simulink model "BergmanModelExtended"  (R2020b)
settings: Solver=VariableStepAuto  StartTime=0.0  StopTime=1000  RelTol=1e-3
undefined symbols (not defined in the file): U1, u3
settings Model: Creator=marti  LastModifiedBy=13234
settings DataIOCC: ReturnWorkspaceOutputs=off
settings DebuggingCC: ArithmeticOperatorsInVariantConditions=warning
settings SFSimCC: CustomCodeUndefinedFunction=UseInterfaceOnly

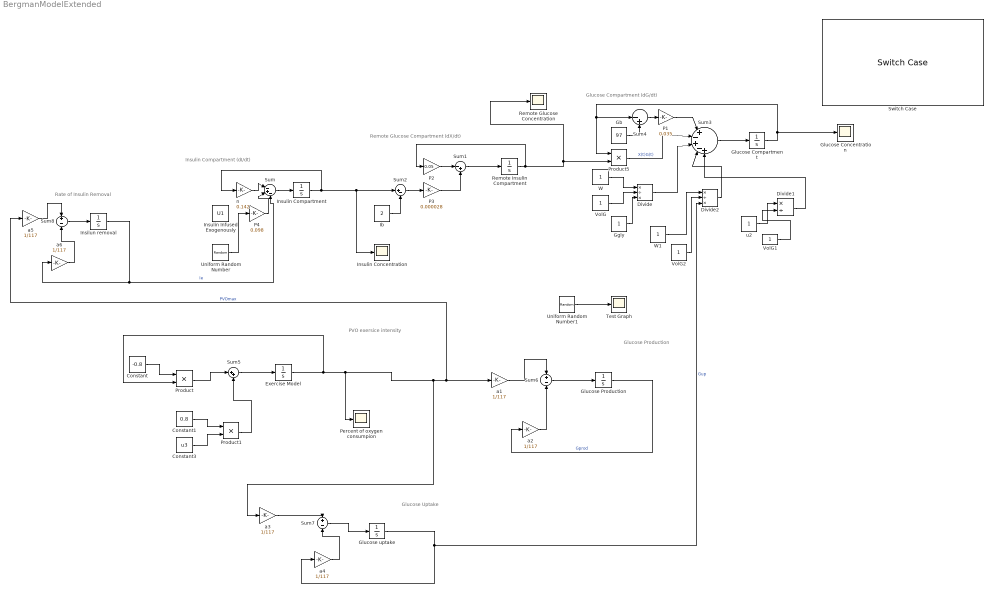
== system BergmanModelExtended ==
  note: Rate of Insulin Removal
  note: Glucose Uptake
  note: Glucose Production
  note: PVO exersice intensity
  note: Insulin Compartment (dI/dt)
  note: Glucose Compartment (dG/dt)
  note: Remote Glucose Compartment (dX/dt)
  Constant : Constant  Value=-0.8
  Constant1 : Constant  Value=0.8
  Constant3 : Constant  Value=u3
  Divide : Product  Inputs=*/*
  Divide1 : Product  Inputs=*/
  Divide2 : Product  Inputs=*/*
  "Exercise Model " : Integrator
  Gb : Constant  Value=97
  Ggly : Constant
  Glucose Compartment : Integrator  InitialCondition=97
  Glucose Concentration : Scope
  Glucose Production : Integrator  InitialCondition=97
  Glucose uptake : Integrator  InitialCondition=97
  Ib : Constant  Value=2
  Insilun removal : Integrator  InitialCondition=97
  Insulin Compartment : Integrator  InitialCondition=1
  Insulin Concentration : Scope
  Insulin Infused Exogenously : Constant  Value=U1  OutMin=0  OutMax=10
  P1 : Gain  Gain=0.035
  P2 : Gain  Gain=0.05
  P3 : Gain  Gain=0.000028
  P4 : Gain  Gain=0.098
  "Percent of oxygen consumpion " : Scope
  Product : Product
  Product1 : Product
  Product5 : Product
  Remote Glucose Concentration : Scope
  Remote Insulin Compartment : Integrator
  Sum : Sum  Inputs=|-+-
  Sum1 : Sum  Inputs=|-+
  Sum2 : Sum  Inputs=|+-
  Sum3 : Sum  Inputs=|+-+-+
  Sum4 : Sum  Inputs=|-+
  Sum5 : Sum  Inputs=|++
  Sum6 : Sum  Inputs=+-
  Sum7 : Sum  Inputs=+-
  Sum8 : Sum  Inputs=+-
  Switch Case : SwitchCase
  Test Graph : Scope
  Uniform Random Number : UniformRandomNumber  Minimum=0  Maximum=10  SampleTime=1
  Uniform Random Number1 : UniformRandomNumber  Minimum=0  Maximum=10  SampleTime=1
  VolG : Constant
  VolG1 : Constant
  VolG2 : Constant
  W : Constant
  W1 : Constant
  a{1..6} (6 alike) : Gain  Gain=1/117
  n : Gain  Gain=0.142
  u2 : Constant
  wires:
  Remote Insulin Compartment/1 -> P2/1, Remote Glucose Concentration/1, Product5/2
  Insulin Compartment/1 -> n/1, Insulin Concentration/1, Sum2/1
  Uniform Random Number1/1 -> Test Graph/1
  Product5/1 -> Sum3/2  "X(t)G(t)"
  P3/1 -> Sum1/2
  Sum1/1 -> Remote Insulin Compartment/1
  Gb/1 -> Sum4/2
  Sum/1 -> Insulin Compartment/1
  P2/1 -> Sum1/1
  Sum3/1 -> Glucose Compartment/1
  P1/1 -> Sum3/1
  Sum4/1 -> P1/1
  Glucose Compartment/1 -> Product5/1, Sum4/1, Glucose Concentration/1
  Sum2/1 -> P3/1
  Uniform Random Number/1 -> P4/1
  Product/1 -> Sum5/1
  Constant/1 -> Product/1
  Constant1/1 -> Product1/1
  Constant3/1 -> Product1/2
  Product1/1 -> Sum5/2
  Sum5/1 -> "Exercise Model "/1
  n/1 -> Sum/1
  P4/1 -> Sum/2
  Ib/1 -> Sum2/2
  "Exercise Model "/1 -> Product/2, "Percent of oxygen consumpion "/1, a3/1, a5/1, a1/1  "PVOmax"
  a1/1 -> Sum6/1
  Sum6/1 -> Glucose Production/1
  a2/1 -> Sum6/2
  Glucose Production/1 -> a2/1  "Gprod"
  a3/1 -> Sum7/1
  Sum7/1 -> Glucose uptake/1
  Glucose uptake/1 -> Divide2/3, a4/1  "Gup"
  a4/1 -> Sum7/2
  a5/1 -> Sum8/1
  Sum8/1 -> Insilun removal/1
  Insilun removal/1 -> a6/1, Sum/3  "Ie"
  a6/1 -> Sum8/2
  W/1 -> Divide/1
  VolG/1 -> Divide/2
  Divide/1 -> Sum3/3
  Ggly/1 -> Divide/3
  u2/1 -> Divide1/1
  VolG1/1 -> Divide1/2
  Divide1/1 -> Sum3/5
  W1/1 -> Divide2/1
  VolG2/1 -> Divide2/2
  Divide2/1 -> Sum3/4
